simulink model "tp2p1demo"  (R2015a)
settings: Solver=ode45  StartTime=0.0  StopTime=350  RelTol=1e-3
undefined symbols (not defined in the file or in its folder): k, k0
settings Model: Creator=Dano  LastModifiedBy=Dano
settings DataIOCC: Refine=10

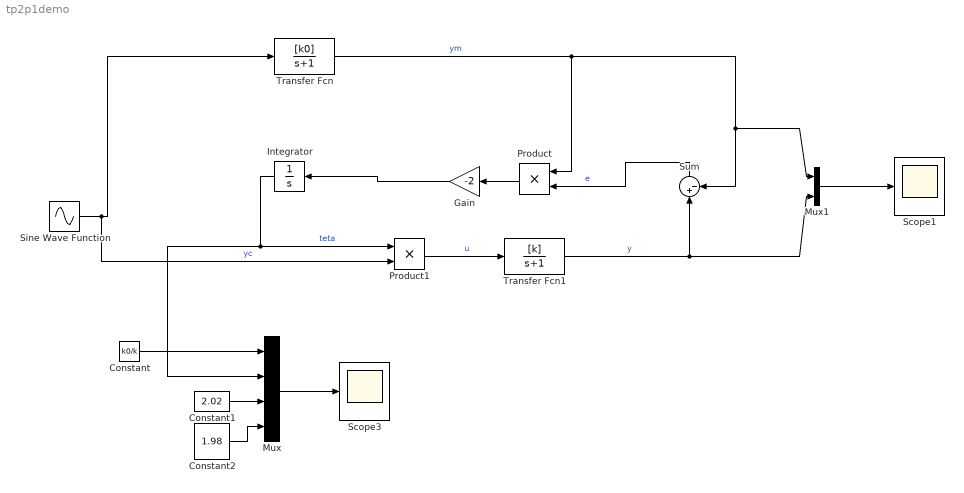
== system tp2p1demo ==
  Constant : Constant  Value=k0/k
  Constant1 : Constant  Value=2.02
  Constant2 : Constant  Value=1.98
  Gain : Gain  Gain=-2
  Integrator : Integrator
  Mux : Mux
  Mux1 : Mux  Inputs=2
  Product : Product
  Product1 : Product
  Scope1 : Scope
  Scope3 : Scope
      settings: SaveName=ScopeData2
  Sine Wave Function : Sin  SampleTime=0
  Sum : Sum  Inputs=|+-
  Transfer Fcn : TransferFcn  Numerator=[k0]  Denominator=[1 1]
  Transfer Fcn1 : TransferFcn  Numerator=[k]  Denominator=[1 1]
  wires:
  Transfer Fcn/1 -> Product/1, Sum/2, Mux1/1  "ym"
  Sum/1 -> Product/2  "e"
  Transfer Fcn1/1 -> Sum/1, Mux1/2  "y"
  Product1/1 -> Transfer Fcn1/1  "u"
  Integrator/1 -> Product1/1, Mux/2  "teta"
  Constant/1 -> Mux/1
  Mux/1 -> Scope3/1
  Product/1 -> Gain/1
  Gain/1 -> Integrator/1
  Sine Wave Function/1 -> Product1/2, Transfer Fcn/1  "yc"
  Mux1/1 -> Scope1/1
  Constant1/1 -> Mux/3
  Constant2/1 -> Mux/4
